simulink model "inverted_pendulum"  (R2015a)
settings: Solver=ode3  StartTime=0.0  StopTime=2  FixedStep=0.001  RelTol=1e-3
values from neighbouring files (symbols this model uses):
  A = -b/m    (= -0.5)    [cruise_control_ss.m]    (also in inverted_pendulum_m.m = [0      1              0           0; inverted_pendulum_simple.m = [0 1; -g/l 0])
  B = 1/m    (= 0.01)    [cruise_control_ss.m]    (also in inverted_pendulum_m.m = [     0; inverted_pendulum_simple.m = [0 g/l]')
  C = 1    [cruise_control_ss.m]    (also in inverted_pendulum_m.m = [1 0 0 0; inverted_pendulum_simple.m = [1 0])
  D = 0    [cruise_control_ss.m]    (also in inverted_pendulum_m.m = [0; inverted_pendulum_simple.m)
settings Model: Creator=Xiaotian  LastModifiedBy=Xiaotian

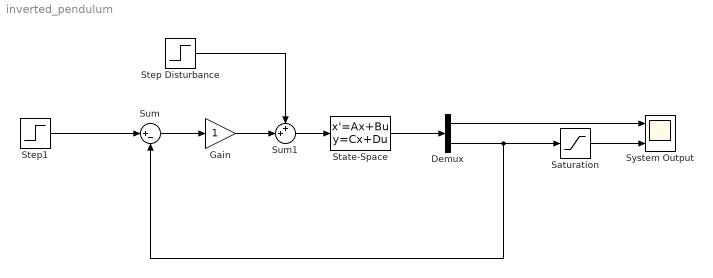
== system inverted_pendulum ==
  Demux : Demux  Outputs=2
  Gain : Gain
  Saturation : Saturate  UpperLimit=1.57  LowerLimit=-1.57
  State-Space : StateSpace  A=A  B=B  C=C  D=D  X0=0
  Step Disturbance : Step  After=0  SampleTime=0
  Step1 : Step  After=0  SampleTime=0
  Sum : Sum  Inputs=|+-
  Sum1 : Sum  Inputs=++|
  System Output : Scope  NumInputPorts=2
      settings: TickLabels=on  TimeRange=10  YMin=0~0  YMax=1.4~1.6  MaxDataPoints=10000
  wires:
  Sum/1 -> Gain/1
  State-Space/1 -> Demux/1
  Demux/1 -> System Output/1
  Saturation/1 -> System Output/2
  Step1/1 -> Sum/1
  Demux/2 -> Sum/2, Saturation/1
  Gain/1 -> Sum1/2
  Sum1/1 -> State-Space/1
  Step Disturbance/1 -> Sum1/1
